simulink model "StdAnimation_Runner"  (R2017b)
settings: configuration reference "VLS_SIL_Configuration" (kept outside this file)
undefined symbols (not defined in the file): C_AnimationPeriod
libraries: simulink x1
settings Model: DataDictionary=Copy_of_StdAnimation_DD_New.sldd  Creator=mchawa  LastModifiedBy=oashraf

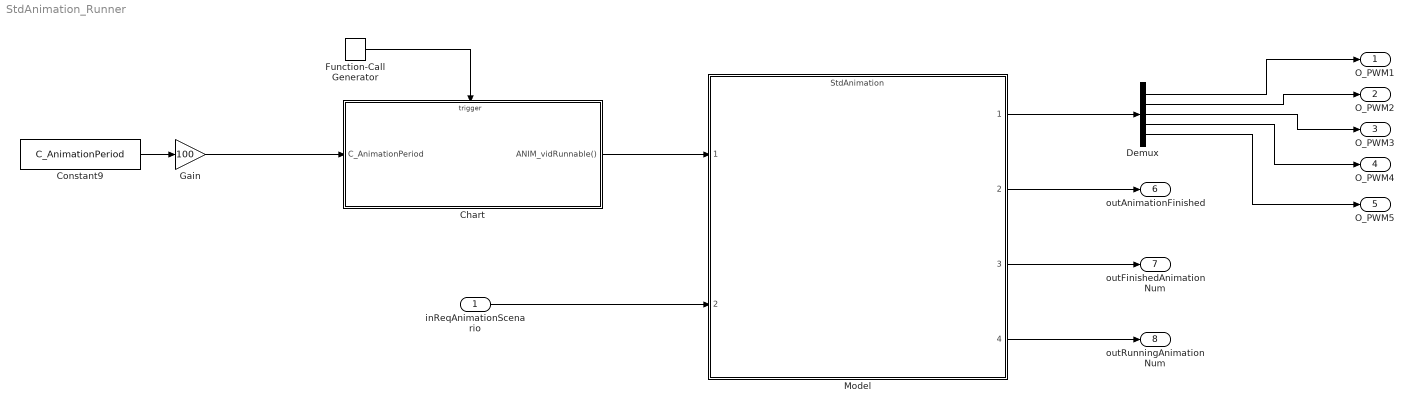
== system StdAnimation_Runner ==
  inReqAnimationScenario : Inport
  Chart : Stateflow chart  TreatAsAtomicUnit=on
  Constant9 : Constant  Value=C_AnimationPeriod
  Demux : Demux  Outputs=5
  Function-Call Generator : simulink/Ports & Subsystems/Function-Call Generator  sample_time=0.01  numberOfIterations=1
  Gain : Gain  Gain=100  OutDataTypeStr=uint8  RndMeth=Round
  Model : ModelReference  ModelNameDialog=StdAnimation.slx  SimulationMode=Normal  ShowModelPeriodicEventPorts=on  ModelReferenceVersion=1.57
  O_PWM1 : Outport
  O_PWM2 : Outport  Port=2
  O_PWM3 : Outport  Port=3
  O_PWM4 : Outport  Port=4
  O_PWM5 : Outport  Port=5
  outAnimationFinished : Outport  Port=6
  outFinishedAnimationNum : Outport  Port=7
  outRunningAnimationNum : Outport  Port=8
  wires:
  Chart/1(ANIM_vidRunnable()) -> Model/1
  Constant9/1 -> Gain/1
  Function-Call Generator/1 -> Chart/Trigger
  Model/2 -> outAnimationFinished/1
  Model/3 -> outFinishedAnimationNum/1
  Model/4 -> outRunningAnimationNum/1
  inReqAnimationScenario/1 -> Model/2
  Demux/3 -> O_PWM3/1
  Demux/2 -> O_PWM2/1
  Demux/4 -> O_PWM4/1
  Demux/1 -> O_PWM1/1
  Demux/5 -> O_PWM5/1
  Gain/1 -> Chart/1(C_AnimationPeriod)
  Model/1 -> Demux/1

== stateflow chart StdAnimation_Runner/Chart ==
  settings: executeAtInitialization=1
  state Scheduler
    on every(C_AnimationPeriod, tik):
    send(ANIM_vidRunnable);
  (default) -> Scheduler
  data: C_AnimationPeriod input
  events: ANIM_vidRunnable output FUNCTION_CALL_EVENT; tik input FUNCTION_CALL_EVENT
